simulink model "poco_ref_al_r307"  (Simulink 6.2)
settings: Solver=ode45  StartTime=0.0  StopTime=100000  RelTol=1e-3
libraries: xbsIndex_r3 x1012, xps_library x42, ddc_library x4, adcscope_lib x2, fft_library x2, pfb_library x2, delay_lib x1
(part 4 of 9)

== system poco_ref_al_r307/delay_wideband_prog0/delay_dp3 ==
  din : Inport  Port=1  LatchInput=off
  delay : Inport  Port=2  LatchInput=off
  AddSub : xbsIndex_r3/AddSub  mode=Subtraction  precision=User Defined  arith_type=Unsigned  n_bits=11  bin_pt=0  quantization=Truncate  overflow=Wrap  latency=1  explicit_period=off  period=1  use_carryin=off  use_carryout=off  en=off  dbl_ovrd=off  show_param=off  use_core=on  pipeline=off  use_rpm=on  gen_core=off
      settings: xl_area=[0, 0, 0, 0, 0, 0, 0]
  Constant2 : xbsIndex_r3/Constant  const=1  equ=P=C  arith_type=Boolean  n_bits=1  bin_pt=0  opselect=C  inp2=PCIN>>17  opr=+  inp1=P  carry=CIN  iostate=0  explicit_period=on  period=1  dbl_ovrd=off
  Constant4 : xbsIndex_r3/Constant  const=0  equ=P=C  arith_type=Boolean  n_bits=1  bin_pt=0  opselect=C  inp2=PCIN>>17  opr=+  inp1=P  carry=CIN  iostate=0  explicit_period=on  period=1  dbl_ovrd=off
  Dual Port RAM : S-Function  AncestorBlock=xbsIndex_r3/Dual Port RAM  FunctionName=xldpram  Parameters=sfcn_mwsv__  mask(Xilinx Dual Port Random Access Memory){depth=2048, initVector=0, write_mode_A=Read After Write, write_mode_B=Read After Write, latency=4, mem_collision=off, init_zero=on, explicit_period=off, period=1, dbl_ovrd=off, rst_a=off, init_a=0, rst_b=off, init_b=0, show_param=off, distributed_mem=off, use_rpm=off, gen_core=off, xl_area=[0, 0, 0, 0, 0, 0, 0], xl_use_area=off}
      mask prompts: initVector "Initial Value Vector"; write_mode_A "Write Mode:  Port A"; write_mode_B "Write Mode:  Port B"; mem_collision "Provide Output Valid Port"; init_zero "Zero Initial Output  (otherwise NaN)"; explicit_period "Use Explicit Sample Period"; period "Sample Period  (use -1 to inherit first known input period)"; dbl_ovrd "Override with Doubles"; rst_a "Provide Reset Port for Port A Output Register"; init_a "Initial Value for Port A Output Register"; rst_b "Provide Reset Port for Port B Output Register"; init_b "Initial Value for Port B Output Register"; show_param "---------------------- Show Implementation Parameters -----------------------------------------------------------------------------------"; distributed_mem "Use Distributed Memory (instead of block RAM)"; use_rpm "Use Placement Information for Core"; gen_core "Generate Core"; xl_area "FPGA Area [Slices, FFs, BRAMs, LUTs, IOBs, Emb. Mults, TBUFs]"; xl_use_area "Use Area Above For Estimation"
      mask help: Dual port random access memory (RAM). Independent address, data and write enable ports allow shared access to a single memory space. Dual ports enable simultaneous access to the memory space at different sample rates using multiple data widths.
      mask init: same as poco_ref_al_r307/delay_wideband_prog0/delay_dp/Dual Port RAM
      mask Help: eval('xlWeb(xlhtmldoclink(''Dual Port RAM''))');
      mask StyleString: edit,edit,popup(Read After Write|Read Before Write|No Read On Write),popup(Read After Write|Read Before Write|No Read On Write),edit,checkbox,checkbox,checkbox,edit,checkbox,checkbox,edit,checkbox,edit,checkbox,checkbox,checkbox,checkbox,edit,checkbox
      mask CallbackString: |||||||xldpramCallback|||xldpramCallback||xldpramCallback||xldpramCallback|xldpramCallback||||
      mask Display:
      | patch([0 iWidth iWidth 0],[0 0 iHeight iHeight] ,bg);
      | patch([0 iWidth iWidth 0],[iCy-2 iCy-2 iCy+2 iCy+2] , .9* bg);
      | patch(logoX,logoY , fg);
      | port_label('input',1,'addr_A');
      | port_label('input',2,'data_A');
      | port_label('input',3,'we_A');
      | port_label('input',4,'addr_B');
      | port_label('input',dataBPNum,dataBStr);
      | port_label('input',weBPNum,weBStr);
      | port_label('input',rstAPNum,rstAStr);
      | port_label('input',rstBPNum,rstBStr);
      | port_label('output',1,'A');
      | port_label('output',doutBPNum,'B');
      | port_label('output',voutAPNum,voutAStr);
      | port_label('output',voutBPNum,voutBStr);
      | ;plot([0 0 iWidth iWidth 0], [0 iHeight iHeight 0 0]);
  wr_addr : xbsIndex_r3/Counter  cnt_type=Free Running  n_bits=11  bin_pt=0  arith_type=Unsigned  start_count=0  cnt_to=Inf  cnt_by_val=1  operation=Up  explicit_period=off  period=1  load_pin=off  rst=off  en=off  dbl_ovrd=off  show_param=off  use_rpm=on  gen_core=off
      settings: xl_area=[0, 0, 0, 0, 0, 0, 0]
  dout : Outport
  wires:
  wr_addr/1 -> AddSub/1, Dual Port RAM/1
  Constant2/1 -> Dual Port RAM/3
  din/1 -> Dual Port RAM/5, Dual Port RAM/2
  Constant4/1 -> Dual Port RAM/6
  delay/1 -> AddSub/2
  AddSub/1 -> Dual Port RAM/4
  Dual Port RAM/2 -> dout/1

== system poco_ref_al_r307/delay_wideband_prog0/sync_delay ==
  In : Inport  Port=1  LatchInput=off
  Constant : xbsIndex_r3/Constant  const=1  equ=P=C  arith_type=Unsigned  n_bits=BitWidth  bin_pt=0  opselect=C  inp2=PCIN>>17  opr=+  inp1=P  carry=CIN  iostate=0  explicit_period=on  period=1  dbl_ovrd=off
  Constant1 : xbsIndex_r3/Constant  const=0  equ=P=C  arith_type=Unsigned  n_bits=BitWidth  bin_pt=0  opselect=C  inp2=PCIN>>17  opr=+  inp1=P  carry=CIN  iostate=0  explicit_period=on  period=1  dbl_ovrd=off
  Constant2 : xbsIndex_r3/Constant  const=DelayLen  equ=P=C  arith_type=Unsigned  n_bits=BitWidth  bin_pt=0  opselect=C  inp2=PCIN>>17  opr=+  inp1=P  carry=CIN  iostate=0  explicit_period=on  period=1  dbl_ovrd=off
  Constant3 : xbsIndex_r3/Constant  const=UseCounter  equ=P=C  arith_type=Unsigned  n_bits=1  bin_pt=0  opselect=C  inp2=PCIN>>17  opr=+  inp1=P  carry=CIN  iostate=0  explicit_period=on  period=1  dbl_ovrd=off
  Counter : xbsIndex_r3/Counter  cnt_type=Free Running  n_bits=BitWidth  bin_pt=0  arith_type=Unsigned  start_count=0  cnt_to=Inf  cnt_by_val=1  operation=Down  explicit_period=on  period=1  load_pin=on  rst=off  en=on  dbl_ovrd=off  show_param=off  use_rpm=on  gen_core=off
      settings: xl_area=[0, 0, 0, 0, 0, 0, 0]
  Logical : xbsIndex_r3/Logical  logical_function=OR  inputs=2  precision=Full  arith_type=Unsigned  n_bits=8  bin_pt=2  align_bp=on  latency=0  explicit_period=on  period=1  en=off  dbl_ovrd=off  show_param=off
      settings: xl_area=[0, 0, 0, 0, 0, 0, 0]
  Mux : xbsIndex_r3/Mux  inputs=2  precision=Full  arith_type="Signed  (2's comp)"  n_bits=8  bin_pt=2  quantization=Truncate  overflow=Wrap  latency=0  explicit_period=off  period=1  en=off  dbl_ovrd=off  show_param=off  mux_type=off  use_rpm=off  gen_core=off
      settings: xl_area=[0, 0, 0, 0, 0, 0, 0]
  Relational : xbsIndex_r3/Relational  mode=a=b  latency=0  explicit_period=off  period=1  en=off  dbl_ovrd=off  show_param=off
      settings: xl_area=[0, 0, 0, 0, 0, 0, 0]
  Relational1 : xbsIndex_r3/Relational  mode=a!=b  latency=0  explicit_period=on  period=1  en=off  dbl_ovrd=off  show_param=off
      settings: xl_area=[0, 0, 0, 0, 0, 0, 0]
  Out : Outport
  wires:
  Counter/1 -> Relational1/1, Relational/2
  Constant1/1 -> Relational1/2
  Constant/1 -> Relational/1
  Constant2/1 -> Counter/2
  In/1 -> Counter/1, Logical/1, Mux/2
  Logical/1 -> Counter/3
  Relational1/1 -> Logical/2
  Relational/1 -> Mux/3
  Constant3/1 -> Mux/1
  Mux/1 -> Out/1

== system poco_ref_al_r307/delay_wideband_prog1/barrel_switcher ==
  sel : Inport  Port=1  LatchInput=off
  sync_in : Inport  Port=2  LatchInput=off
  In1 : Inport  Port=3  LatchInput=off
  In2 : Inport  Port=4  LatchInput=off
  In3 : Inport  Port=5  LatchInput=off
  In4 : Inport  Port=6  LatchInput=off
  Delay1 : xbsIndex_r3/Delay  latency=1  reg_retiming=off  explicit_period=off  period=1  en=off  accept_only_valid=off  init_zero=on  dbl_ovrd=off  show_param=off
      settings: xl_area=[0, 0, 0, 0, 0, 0, 0]
  Delay_sync : xbsIndex_r3/Delay  latency=2  reg_retiming=off  explicit_period=off  period=1  en=off  accept_only_valid=off  init_zero=on  dbl_ovrd=off  show_param=off
      settings: xl_area=[0, 0, 0, 0, 0, 0, 0]
  Mux{11..12,21..22,31..32,41..42} (8 alike) : xbsIndex_r3/Mux  inputs=2  precision=Full  arith_type="Signed  (2's comp)"  n_bits=8  bin_pt=2  quantization=Truncate  overflow=Wrap  latency=1  explicit_period=off  period=1  en=off  dbl_ovrd=off  show_param=off  mux_type=off  use_rpm=off  gen_core=off
      settings: xl_area=[0, 0, 0, 0, 0, 0, 0]
  Slice1 : xbsIndex_r3/Slice  mode=Upper Bit Location + Width  nbits=1  bit1=-0  base1=MSB of Input  bit0=0  base0=LSB of Input  boolean_output=off  explicit_period=off  period=1  dbl_ovrd=off
  Slice2 : xbsIndex_r3/Slice  mode=Upper Bit Location + Width  nbits=1  bit1=-1  base1=MSB of Input  bit0=0  base0=LSB of Input  boolean_output=off  explicit_period=off  period=1  dbl_ovrd=off
  sync_out : Outport
  Out1 : Outport  Port=2
  Out2 : Outport  Port=3
  Out3 : Outport  Port=4
  Out4 : Outport  Port=5
  wires:
  Mux41/1 -> Mux32/3, Mux42/2
  Mux31/1 -> Mux22/3, Mux32/2
  Mux21/1 -> Mux12/3, Mux22/2
  Mux11/1 -> Mux42/3, Mux12/2
  Mux42/1 -> Out4/1
  In4/1 -> Mux21/3, Mux41/2
  Mux32/1 -> Out3/1
  In3/1 -> Mux11/3, Mux31/2
  Mux22/1 -> Out2/1
  In2/1 -> Mux41/3, Mux21/2
  Mux12/1 -> Out1/1
  In1/1 -> Mux31/3, Mux11/2
  Slice2/1 -> Mux42/1, Mux32/1, Mux22/1, Mux12/1
  Slice1/1 -> Mux41/1, Mux31/1, Mux21/1, Mux11/1
  Delay1/1 -> Slice2/1
  sel/1 -> Delay1/1, Slice1/1
  Delay_sync/1 -> sync_out/1
  sync_in/1 -> Delay_sync/1

== system poco_ref_al_r307/delay_wideband_prog1/delay_dp ==
  din : Inport  Port=1  LatchInput=off
  delay : Inport  Port=2  LatchInput=off
  AddSub : xbsIndex_r3/AddSub  mode=Subtraction  precision=User Defined  arith_type=Unsigned  n_bits=11  bin_pt=0  quantization=Truncate  overflow=Wrap  latency=1  explicit_period=off  period=1  use_carryin=off  use_carryout=off  en=off  dbl_ovrd=off  show_param=off  use_core=on  pipeline=off  use_rpm=on  gen_core=off
      settings: xl_area=[0, 0, 0, 0, 0, 0, 0]
  Constant2 : xbsIndex_r3/Constant  const=1  equ=P=C  arith_type=Boolean  n_bits=1  bin_pt=0  opselect=C  inp2=PCIN>>17  opr=+  inp1=P  carry=CIN  iostate=0  explicit_period=on  period=1  dbl_ovrd=off
  Constant4 : xbsIndex_r3/Constant  const=0  equ=P=C  arith_type=Boolean  n_bits=1  bin_pt=0  opselect=C  inp2=PCIN>>17  opr=+  inp1=P  carry=CIN  iostate=0  explicit_period=on  period=1  dbl_ovrd=off
  Dual Port RAM : S-Function  AncestorBlock=xbsIndex_r3/Dual Port RAM  FunctionName=xldpram  Parameters=sfcn_mwsv__  mask(Xilinx Dual Port Random Access Memory){depth=2048, initVector=0, write_mode_A=Read After Write, write_mode_B=Read After Write, latency=4, mem_collision=off, init_zero=on, explicit_period=off, period=1, dbl_ovrd=off, rst_a=off, init_a=0, rst_b=off, init_b=0, show_param=off, distributed_mem=off, use_rpm=off, gen_core=off, xl_area=[0, 0, 0, 0, 0, 0, 0], xl_use_area=off}
      mask prompts: initVector "Initial Value Vector"; write_mode_A "Write Mode:  Port A"; write_mode_B "Write Mode:  Port B"; mem_collision "Provide Output Valid Port"; init_zero "Zero Initial Output  (otherwise NaN)"; explicit_period "Use Explicit Sample Period"; period "Sample Period  (use -1 to inherit first known input period)"; dbl_ovrd "Override with Doubles"; rst_a "Provide Reset Port for Port A Output Register"; init_a "Initial Value for Port A Output Register"; rst_b "Provide Reset Port for Port B Output Register"; init_b "Initial Value for Port B Output Register"; show_param "---------------------- Show Implementation Parameters -----------------------------------------------------------------------------------"; distributed_mem "Use Distributed Memory (instead of block RAM)"; use_rpm "Use Placement Information for Core"; gen_core "Generate Core"; xl_area "FPGA Area [Slices, FFs, BRAMs, LUTs, IOBs, Emb. Mults, TBUFs]"; xl_use_area "Use Area Above For Estimation"
      mask help: Dual port random access memory (RAM). Independent address, data and write enable ports allow shared access to a single memory space. Dual ports enable simultaneous access to the memory space at different sample rates using multiple data widths.
      mask init: same as poco_ref_al_r307/delay_wideband_prog0/delay_dp/Dual Port RAM
      mask Help: eval('xlWeb(xlhtmldoclink(''Dual Port RAM''))');
      mask StyleString: edit,edit,popup(Read After Write|Read Before Write|No Read On Write),popup(Read After Write|Read Before Write|No Read On Write),edit,checkbox,checkbox,checkbox,edit,checkbox,checkbox,edit,checkbox,edit,checkbox,checkbox,checkbox,checkbox,edit,checkbox
      mask CallbackString: |||||||xldpramCallback|||xldpramCallback||xldpramCallback||xldpramCallback|xldpramCallback||||
      mask Display:
      | patch([0 iWidth iWidth 0],[0 0 iHeight iHeight] ,bg);
      | patch([0 iWidth iWidth 0],[iCy-2 iCy-2 iCy+2 iCy+2] , .9* bg);
      | patch(logoX,logoY , fg);
      | port_label('input',1,'addr_A');
      | port_label('input',2,'data_A');
      | port_label('input',3,'we_A');
      | port_label('input',4,'addr_B');
      | port_label('input',dataBPNum,dataBStr);
      | port_label('input',weBPNum,weBStr);
      | port_label('input',rstAPNum,rstAStr);
      | port_label('input',rstBPNum,rstBStr);
      | port_label('output',1,'A');
      | port_label('output',doutBPNum,'B');
      | port_label('output',voutAPNum,voutAStr);
      | port_label('output',voutBPNum,voutBStr);
      | ;plot([0 0 iWidth iWidth 0], [0 iHeight iHeight 0 0]);
  wr_addr : xbsIndex_r3/Counter  cnt_type=Free Running  n_bits=11  bin_pt=0  arith_type=Unsigned  start_count=0  cnt_to=Inf  cnt_by_val=1  operation=Up  explicit_period=off  period=1  load_pin=off  rst=off  en=off  dbl_ovrd=off  show_param=off  use_rpm=on  gen_core=off
      settings: xl_area=[0, 0, 0, 0, 0, 0, 0]
  dout : Outport
  wires:
  wr_addr/1 -> AddSub/1, Dual Port RAM/1
  Constant2/1 -> Dual Port RAM/3
  din/1 -> Dual Port RAM/5, Dual Port RAM/2
  Constant4/1 -> Dual Port RAM/6
  delay/1 -> AddSub/2
  AddSub/1 -> Dual Port RAM/4
  Dual Port RAM/2 -> dout/1

== system poco_ref_al_r307/delay_wideband_prog1/delay_dp1 ==
  din : Inport  Port=1  LatchInput=off
  delay : Inport  Port=2  LatchInput=off
  AddSub : xbsIndex_r3/AddSub  mode=Subtraction  precision=User Defined  arith_type=Unsigned  n_bits=11  bin_pt=0  quantization=Truncate  overflow=Wrap  latency=1  explicit_period=off  period=1  use_carryin=off  use_carryout=off  en=off  dbl_ovrd=off  show_param=off  use_core=on  pipeline=off  use_rpm=on  gen_core=off
      settings: xl_area=[0, 0, 0, 0, 0, 0, 0]
  Constant2 : xbsIndex_r3/Constant  const=1  equ=P=C  arith_type=Boolean  n_bits=1  bin_pt=0  opselect=C  inp2=PCIN>>17  opr=+  inp1=P  carry=CIN  iostate=0  explicit_period=on  period=1  dbl_ovrd=off
  Constant4 : xbsIndex_r3/Constant  const=0  equ=P=C  arith_type=Boolean  n_bits=1  bin_pt=0  opselect=C  inp2=PCIN>>17  opr=+  inp1=P  carry=CIN  iostate=0  explicit_period=on  period=1  dbl_ovrd=off
  Dual Port RAM : S-Function  AncestorBlock=xbsIndex_r3/Dual Port RAM  FunctionName=xldpram  Parameters=sfcn_mwsv__  mask(Xilinx Dual Port Random Access Memory){depth=2048, initVector=0, write_mode_A=Read After Write, write_mode_B=Read After Write, latency=4, mem_collision=off, init_zero=on, explicit_period=off, period=1, dbl_ovrd=off, rst_a=off, init_a=0, rst_b=off, init_b=0, show_param=off, distributed_mem=off, use_rpm=off, gen_core=off, xl_area=[0, 0, 0, 0, 0, 0, 0], xl_use_area=off}
      mask prompts: initVector "Initial Value Vector"; write_mode_A "Write Mode:  Port A"; write_mode_B "Write Mode:  Port B"; mem_collision "Provide Output Valid Port"; init_zero "Zero Initial Output  (otherwise NaN)"; explicit_period "Use Explicit Sample Period"; period "Sample Period  (use -1 to inherit first known input period)"; dbl_ovrd "Override with Doubles"; rst_a "Provide Reset Port for Port A Output Register"; init_a "Initial Value for Port A Output Register"; rst_b "Provide Reset Port for Port B Output Register"; init_b "Initial Value for Port B Output Register"; show_param "---------------------- Show Implementation Parameters -----------------------------------------------------------------------------------"; distributed_mem "Use Distributed Memory (instead of block RAM)"; use_rpm "Use Placement Information for Core"; gen_core "Generate Core"; xl_area "FPGA Area [Slices, FFs, BRAMs, LUTs, IOBs, Emb. Mults, TBUFs]"; xl_use_area "Use Area Above For Estimation"
      mask help: Dual port random access memory (RAM). Independent address, data and write enable ports allow shared access to a single memory space. Dual ports enable simultaneous access to the memory space at different sample rates using multiple data widths.
      mask init: same as poco_ref_al_r307/delay_wideband_prog0/delay_dp/Dual Port RAM
      mask Help: eval('xlWeb(xlhtmldoclink(''Dual Port RAM''))');
      mask StyleString: edit,edit,popup(Read After Write|Read Before Write|No Read On Write),popup(Read After Write|Read Before Write|No Read On Write),edit,checkbox,checkbox,checkbox,edit,checkbox,checkbox,edit,checkbox,edit,checkbox,checkbox,checkbox,checkbox,edit,checkbox
      mask CallbackString: |||||||xldpramCallback|||xldpramCallback||xldpramCallback||xldpramCallback|xldpramCallback||||
      mask Display:
      | patch([0 iWidth iWidth 0],[0 0 iHeight iHeight] ,bg);
      | patch([0 iWidth iWidth 0],[iCy-2 iCy-2 iCy+2 iCy+2] , .9* bg);
      | patch(logoX,logoY , fg);
      | port_label('input',1,'addr_A');
      | port_label('input',2,'data_A');
      | port_label('input',3,'we_A');
      | port_label('input',4,'addr_B');
      | port_label('input',dataBPNum,dataBStr);
      | port_label('input',weBPNum,weBStr);
      | port_label('input',rstAPNum,rstAStr);
      | port_label('input',rstBPNum,rstBStr);
      | port_label('output',1,'A');
      | port_label('output',doutBPNum,'B');
      | port_label('output',voutAPNum,voutAStr);
      | port_label('output',voutBPNum,voutBStr);
      | ;plot([0 0 iWidth iWidth 0], [0 iHeight iHeight 0 0]);
  wr_addr : xbsIndex_r3/Counter  cnt_type=Free Running  n_bits=11  bin_pt=0  arith_type=Unsigned  start_count=0  cnt_to=Inf  cnt_by_val=1  operation=Up  explicit_period=off  period=1  load_pin=off  rst=off  en=off  dbl_ovrd=off  show_param=off  use_rpm=on  gen_core=off
      settings: xl_area=[0, 0, 0, 0, 0, 0, 0]
  dout : Outport
  wires:
  Dual Port RAM/2 -> dout/1
  AddSub/1 -> Dual Port RAM/4
  delay/1 -> AddSub/2
  Constant4/1 -> Dual Port RAM/6
  din/1 -> Dual Port RAM/2, Dual Port RAM/5
  Constant2/1 -> Dual Port RAM/3
  wr_addr/1 -> Dual Port RAM/1, AddSub/1

== system poco_ref_al_r307/delay_wideband_prog1/delay_dp2 ==
  din : Inport  Port=1  LatchInput=off
  delay : Inport  Port=2  LatchInput=off
  AddSub : xbsIndex_r3/AddSub  mode=Subtraction  precision=User Defined  arith_type=Unsigned  n_bits=11  bin_pt=0  quantization=Truncate  overflow=Wrap  latency=1  explicit_period=off  period=1  use_carryin=off  use_carryout=off  en=off  dbl_ovrd=off  show_param=off  use_core=on  pipeline=off  use_rpm=on  gen_core=off
      settings: xl_area=[0, 0, 0, 0, 0, 0, 0]
  Constant2 : xbsIndex_r3/Constant  const=1  equ=P=C  arith_type=Boolean  n_bits=1  bin_pt=0  opselect=C  inp2=PCIN>>17  opr=+  inp1=P  carry=CIN  iostate=0  explicit_period=on  period=1  dbl_ovrd=off
  Constant4 : xbsIndex_r3/Constant  const=0  equ=P=C  arith_type=Boolean  n_bits=1  bin_pt=0  opselect=C  inp2=PCIN>>17  opr=+  inp1=P  carry=CIN  iostate=0  explicit_period=on  period=1  dbl_ovrd=off
  Dual Port RAM : S-Function  AncestorBlock=xbsIndex_r3/Dual Port RAM  FunctionName=xldpram  Parameters=sfcn_mwsv__  mask(Xilinx Dual Port Random Access Memory){depth=2048, initVector=0, write_mode_A=Read After Write, write_mode_B=Read After Write, latency=4, mem_collision=off, init_zero=on, explicit_period=off, period=1, dbl_ovrd=off, rst_a=off, init_a=0, rst_b=off, init_b=0, show_param=off, distributed_mem=off, use_rpm=off, gen_core=off, xl_area=[0, 0, 0, 0, 0, 0, 0], xl_use_area=off}
      mask prompts: initVector "Initial Value Vector"; write_mode_A "Write Mode:  Port A"; write_mode_B "Write Mode:  Port B"; mem_collision "Provide Output Valid Port"; init_zero "Zero Initial Output  (otherwise NaN)"; explicit_period "Use Explicit Sample Period"; period "Sample Period  (use -1 to inherit first known input period)"; dbl_ovrd "Override with Doubles"; rst_a "Provide Reset Port for Port A Output Register"; init_a "Initial Value for Port A Output Register"; rst_b "Provide Reset Port for Port B Output Register"; init_b "Initial Value for Port B Output Register"; show_param "---------------------- Show Implementation Parameters -----------------------------------------------------------------------------------"; distributed_mem "Use Distributed Memory (instead of block RAM)"; use_rpm "Use Placement Information for Core"; gen_core "Generate Core"; xl_area "FPGA Area [Slices, FFs, BRAMs, LUTs, IOBs, Emb. Mults, TBUFs]"; xl_use_area "Use Area Above For Estimation"
      mask help: Dual port random access memory (RAM). Independent address, data and write enable ports allow shared access to a single memory space. Dual ports enable simultaneous access to the memory space at different sample rates using multiple data widths.
      mask init: same as poco_ref_al_r307/delay_wideband_prog0/delay_dp/Dual Port RAM
      mask Help: eval('xlWeb(xlhtmldoclink(''Dual Port RAM''))');
      mask StyleString: edit,edit,popup(Read After Write|Read Before Write|No Read On Write),popup(Read After Write|Read Before Write|No Read On Write),edit,checkbox,checkbox,checkbox,edit,checkbox,checkbox,edit,checkbox,edit,checkbox,checkbox,checkbox,checkbox,edit,checkbox
      mask CallbackString: |||||||xldpramCallback|||xldpramCallback||xldpramCallback||xldpramCallback|xldpramCallback||||
      mask Display:
      | patch([0 iWidth iWidth 0],[0 0 iHeight iHeight] ,bg);
      | patch([0 iWidth iWidth 0],[iCy-2 iCy-2 iCy+2 iCy+2] , .9* bg);
      | patch(logoX,logoY , fg);
      | port_label('input',1,'addr_A');
      | port_label('input',2,'data_A');
      | port_label('input',3,'we_A');
      | port_label('input',4,'addr_B');
      | port_label('input',dataBPNum,dataBStr);
      | port_label('input',weBPNum,weBStr);
      | port_label('input',rstAPNum,rstAStr);
      | port_label('input',rstBPNum,rstBStr);
      | port_label('output',1,'A');
      | port_label('output',doutBPNum,'B');
      | port_label('output',voutAPNum,voutAStr);
      | port_label('output',voutBPNum,voutBStr);
      | ;plot([0 0 iWidth iWidth 0], [0 iHeight iHeight 0 0]);
  wr_addr : xbsIndex_r3/Counter  cnt_type=Free Running  n_bits=11  bin_pt=0  arith_type=Unsigned  start_count=0  cnt_to=Inf  cnt_by_val=1  operation=Up  explicit_period=off  period=1  load_pin=off  rst=off  en=off  dbl_ovrd=off  show_param=off  use_rpm=on  gen_core=off
      settings: xl_area=[0, 0, 0, 0, 0, 0, 0]
  dout : Outport
  wires:
  wr_addr/1 -> AddSub/1, Dual Port RAM/1
  Constant2/1 -> Dual Port RAM/3
  din/1 -> Dual Port RAM/5, Dual Port RAM/2
  Constant4/1 -> Dual Port RAM/6
  delay/1 -> AddSub/2
  AddSub/1 -> Dual Port RAM/4
  Dual Port RAM/2 -> dout/1

== system poco_ref_al_r307/delay_wideband_prog1/delay_dp3 ==
  din : Inport  Port=1  LatchInput=off
  delay : Inport  Port=2  LatchInput=off
  AddSub : xbsIndex_r3/AddSub  mode=Subtraction  precision=User Defined  arith_type=Unsigned  n_bits=11  bin_pt=0  quantization=Truncate  overflow=Wrap  latency=1  explicit_period=off  period=1  use_carryin=off  use_carryout=off  en=off  dbl_ovrd=off  show_param=off  use_core=on  pipeline=off  use_rpm=on  gen_core=off
      settings: xl_area=[0, 0, 0, 0, 0, 0, 0]
  Constant2 : xbsIndex_r3/Constant  const=1  equ=P=C  arith_type=Boolean  n_bits=1  bin_pt=0  opselect=C  inp2=PCIN>>17  opr=+  inp1=P  carry=CIN  iostate=0  explicit_period=on  period=1  dbl_ovrd=off
  Constant4 : xbsIndex_r3/Constant  const=0  equ=P=C  arith_type=Boolean  n_bits=1  bin_pt=0  opselect=C  inp2=PCIN>>17  opr=+  inp1=P  carry=CIN  iostate=0  explicit_period=on  period=1  dbl_ovrd=off
  Dual Port RAM : S-Function  AncestorBlock=xbsIndex_r3/Dual Port RAM  FunctionName=xldpram  Parameters=sfcn_mwsv__  mask(Xilinx Dual Port Random Access Memory){depth=2048, initVector=0, write_mode_A=Read After Write, write_mode_B=Read After Write, latency=4, mem_collision=off, init_zero=on, explicit_period=off, period=1, dbl_ovrd=off, rst_a=off, init_a=0, rst_b=off, init_b=0, show_param=off, distributed_mem=off, use_rpm=off, gen_core=off, xl_area=[0, 0, 0, 0, 0, 0, 0], xl_use_area=off}
      mask prompts: initVector "Initial Value Vector"; write_mode_A "Write Mode:  Port A"; write_mode_B "Write Mode:  Port B"; mem_collision "Provide Output Valid Port"; init_zero "Zero Initial Output  (otherwise NaN)"; explicit_period "Use Explicit Sample Period"; period "Sample Period  (use -1 to inherit first known input period)"; dbl_ovrd "Override with Doubles"; rst_a "Provide Reset Port for Port A Output Register"; init_a "Initial Value for Port A Output Register"; rst_b "Provide Reset Port for Port B Output Register"; init_b "Initial Value for Port B Output Register"; show_param "---------------------- Show Implementation Parameters -----------------------------------------------------------------------------------"; distributed_mem "Use Distributed Memory (instead of block RAM)"; use_rpm "Use Placement Information for Core"; gen_core "Generate Core"; xl_area "FPGA Area [Slices, FFs, BRAMs, LUTs, IOBs, Emb. Mults, TBUFs]"; xl_use_area "Use Area Above For Estimation"
      mask help: Dual port random access memory (RAM). Independent address, data and write enable ports allow shared access to a single memory space. Dual ports enable simultaneous access to the memory space at different sample rates using multiple data widths.
      mask init: same as poco_ref_al_r307/delay_wideband_prog0/delay_dp/Dual Port RAM
      mask Help: eval('xlWeb(xlhtmldoclink(''Dual Port RAM''))');
      mask StyleString: edit,edit,popup(Read After Write|Read Before Write|No Read On Write),popup(Read After Write|Read Before Write|No Read On Write),edit,checkbox,checkbox,checkbox,edit,checkbox,checkbox,edit,checkbox,edit,checkbox,checkbox,checkbox,checkbox,edit,checkbox
      mask CallbackString: |||||||xldpramCallback|||xldpramCallback||xldpramCallback||xldpramCallback|xldpramCallback||||
      mask Display:
      | patch([0 iWidth iWidth 0],[0 0 iHeight iHeight] ,bg);
      | patch([0 iWidth iWidth 0],[iCy-2 iCy-2 iCy+2 iCy+2] , .9* bg);
      | patch(logoX,logoY , fg);
      | port_label('input',1,'addr_A');
      | port_label('input',2,'data_A');
      | port_label('input',3,'we_A');
      | port_label('input',4,'addr_B');
      | port_label('input',dataBPNum,dataBStr);
      | port_label('input',weBPNum,weBStr);
      | port_label('input',rstAPNum,rstAStr);
      | port_label('input',rstBPNum,rstBStr);
      | port_label('output',1,'A');
      | port_label('output',doutBPNum,'B');
      | port_label('output',voutAPNum,voutAStr);
      | port_label('output',voutBPNum,voutBStr);
      | ;plot([0 0 iWidth iWidth 0], [0 iHeight iHeight 0 0]);
  wr_addr : xbsIndex_r3/Counter  cnt_type=Free Running  n_bits=11  bin_pt=0  arith_type=Unsigned  start_count=0  cnt_to=Inf  cnt_by_val=1  operation=Up  explicit_period=off  period=1  load_pin=off  rst=off  en=off  dbl_ovrd=off  show_param=off  use_rpm=on  gen_core=off
      settings: xl_area=[0, 0, 0, 0, 0, 0, 0]
  dout : Outport
  wires:
  Dual Port RAM/2 -> dout/1
  AddSub/1 -> Dual Port RAM/4
  delay/1 -> AddSub/2
  Constant4/1 -> Dual Port RAM/6
  din/1 -> Dual Port RAM/2, Dual Port RAM/5
  Constant2/1 -> Dual Port RAM/3
  wr_addr/1 -> Dual Port RAM/1, AddSub/1

== system poco_ref_al_r307/delay_wideband_prog1/sync_delay ==
  In : Inport  Port=1  LatchInput=off
  Constant : xbsIndex_r3/Constant  const=1  equ=P=C  arith_type=Unsigned  n_bits=BitWidth  bin_pt=0  opselect=C  inp2=PCIN>>17  opr=+  inp1=P  carry=CIN  iostate=0  explicit_period=on  period=1  dbl_ovrd=off
  Constant1 : xbsIndex_r3/Constant  const=0  equ=P=C  arith_type=Unsigned  n_bits=BitWidth  bin_pt=0  opselect=C  inp2=PCIN>>17  opr=+  inp1=P  carry=CIN  iostate=0  explicit_period=on  period=1  dbl_ovrd=off
  Constant2 : xbsIndex_r3/Constant  const=DelayLen  equ=P=C  arith_type=Unsigned  n_bits=BitWidth  bin_pt=0  opselect=C  inp2=PCIN>>17  opr=+  inp1=P  carry=CIN  iostate=0  explicit_period=on  period=1  dbl_ovrd=off
  Constant3 : xbsIndex_r3/Constant  const=UseCounter  equ=P=C  arith_type=Unsigned  n_bits=1  bin_pt=0  opselect=C  inp2=PCIN>>17  opr=+  inp1=P  carry=CIN  iostate=0  explicit_period=on  period=1  dbl_ovrd=off
  Counter : xbsIndex_r3/Counter  cnt_type=Free Running  n_bits=BitWidth  bin_pt=0  arith_type=Unsigned  start_count=0  cnt_to=Inf  cnt_by_val=1  operation=Down  explicit_period=on  period=1  load_pin=on  rst=off  en=on  dbl_ovrd=off  show_param=off  use_rpm=on  gen_core=off
      settings: xl_area=[0, 0, 0, 0, 0, 0, 0]
  Logical : xbsIndex_r3/Logical  logical_function=OR  inputs=2  precision=Full  arith_type=Unsigned  n_bits=8  bin_pt=2  align_bp=on  latency=0  explicit_period=on  period=1  en=off  dbl_ovrd=off  show_param=off
      settings: xl_area=[0, 0, 0, 0, 0, 0, 0]
  Mux : xbsIndex_r3/Mux  inputs=2  precision=Full  arith_type="Signed  (2's comp)"  n_bits=8  bin_pt=2  quantization=Truncate  overflow=Wrap  latency=0  explicit_period=off  period=1  en=off  dbl_ovrd=off  show_param=off  mux_type=off  use_rpm=off  gen_core=off
      settings: xl_area=[0, 0, 0, 0, 0, 0, 0]
  Relational : xbsIndex_r3/Relational  mode=a=b  latency=0  explicit_period=off  period=1  en=off  dbl_ovrd=off  show_param=off
      settings: xl_area=[0, 0, 0, 0, 0, 0, 0]
  Relational1 : xbsIndex_r3/Relational  mode=a!=b  latency=0  explicit_period=on  period=1  en=off  dbl_ovrd=off  show_param=off
      settings: xl_area=[0, 0, 0, 0, 0, 0, 0]
  Out : Outport
  wires:
  Mux/1 -> Out/1
  Constant3/1 -> Mux/1
  Relational/1 -> Mux/3
  Relational1/1 -> Logical/2
  Logical/1 -> Counter/3
  In/1 -> Mux/2, Logical/1, Counter/1
  Constant2/1 -> Counter/2
  Constant/1 -> Relational/1
  Constant1/1 -> Relational1/2
  Counter/1 -> Relational/2, Relational1/1

== system poco_ref_al_r307/delay_wideband_prog2/barrel_switcher ==
  sel : Inport  Port=1  LatchInput=off
  sync_in : Inport  Port=2  LatchInput=off
  In1 : Inport  Port=3  LatchInput=off
  In2 : Inport  Port=4  LatchInput=off
  In3 : Inport  Port=5  LatchInput=off
  In4 : Inport  Port=6  LatchInput=off
  Delay1 : xbsIndex_r3/Delay  latency=1  reg_retiming=off  explicit_period=off  period=1  en=off  accept_only_valid=off  init_zero=on  dbl_ovrd=off  show_param=off
      settings: xl_area=[0, 0, 0, 0, 0, 0, 0]
  Delay_sync : xbsIndex_r3/Delay  latency=2  reg_retiming=off  explicit_period=off  period=1  en=off  accept_only_valid=off  init_zero=on  dbl_ovrd=off  show_param=off
      settings: xl_area=[0, 0, 0, 0, 0, 0, 0]
  Mux{11..12,21..22,31..32,41..42} (8 alike) : xbsIndex_r3/Mux  inputs=2  precision=Full  arith_type="Signed  (2's comp)"  n_bits=8  bin_pt=2  quantization=Truncate  overflow=Wrap  latency=1  explicit_period=off  period=1  en=off  dbl_ovrd=off  show_param=off  mux_type=off  use_rpm=off  gen_core=off
      settings: xl_area=[0, 0, 0, 0, 0, 0, 0]
  Slice1 : xbsIndex_r3/Slice  mode=Upper Bit Location + Width  nbits=1  bit1=-0  base1=MSB of Input  bit0=0  base0=LSB of Input  boolean_output=off  explicit_period=off  period=1  dbl_ovrd=off
  Slice2 : xbsIndex_r3/Slice  mode=Upper Bit Location + Width  nbits=1  bit1=-1  base1=MSB of Input  bit0=0  base0=LSB of Input  boolean_output=off  explicit_period=off  period=1  dbl_ovrd=off
  sync_out : Outport
  Out1 : Outport  Port=2
  Out2 : Outport  Port=3
  Out3 : Outport  Port=4
  Out4 : Outport  Port=5
  wires:
  sync_in/1 -> Delay_sync/1
  Delay_sync/1 -> sync_out/1
  sel/1 -> Slice1/1, Delay1/1
  Delay1/1 -> Slice2/1
  Slice1/1 -> Mux11/1, Mux21/1, Mux31/1, Mux41/1
  Slice2/1 -> Mux12/1, Mux22/1, Mux32/1, Mux42/1
  In1/1 -> Mux11/2, Mux31/3
  Mux12/1 -> Out1/1
  In2/1 -> Mux21/2, Mux41/3
  Mux22/1 -> Out2/1
  In3/1 -> Mux31/2, Mux11/3
  Mux32/1 -> Out3/1
  In4/1 -> Mux41/2, Mux21/3
  Mux42/1 -> Out4/1
  Mux11/1 -> Mux12/2, Mux42/3
  Mux21/1 -> Mux22/2, Mux12/3
  Mux31/1 -> Mux32/2, Mux22/3
  Mux41/1 -> Mux42/2, Mux32/3

== system poco_ref_al_r307/delay_wideband_prog2/delay_dp ==
  din : Inport  Port=1  LatchInput=off
  delay : Inport  Port=2  LatchInput=off
  AddSub : xbsIndex_r3/AddSub  mode=Subtraction  precision=User Defined  arith_type=Unsigned  n_bits=11  bin_pt=0  quantization=Truncate  overflow=Wrap  latency=1  explicit_period=off  period=1  use_carryin=off  use_carryout=off  en=off  dbl_ovrd=off  show_param=off  use_core=on  pipeline=off  use_rpm=on  gen_core=off
      settings: xl_area=[0, 0, 0, 0, 0, 0, 0]
  Constant2 : xbsIndex_r3/Constant  const=1  equ=P=C  arith_type=Boolean  n_bits=1  bin_pt=0  opselect=C  inp2=PCIN>>17  opr=+  inp1=P  carry=CIN  iostate=0  explicit_period=on  period=1  dbl_ovrd=off
  Constant4 : xbsIndex_r3/Constant  const=0  equ=P=C  arith_type=Boolean  n_bits=1  bin_pt=0  opselect=C  inp2=PCIN>>17  opr=+  inp1=P  carry=CIN  iostate=0  explicit_period=on  period=1  dbl_ovrd=off
  Dual Port RAM : S-Function  AncestorBlock=xbsIndex_r3/Dual Port RAM  FunctionName=xldpram  Parameters=sfcn_mwsv__  mask(Xilinx Dual Port Random Access Memory){depth=2048, initVector=0, write_mode_A=Read After Write, write_mode_B=Read After Write, latency=4, mem_collision=off, init_zero=on, explicit_period=off, period=1, dbl_ovrd=off, rst_a=off, init_a=0, rst_b=off, init_b=0, show_param=off, distributed_mem=off, use_rpm=off, gen_core=off, xl_area=[0, 0, 0, 0, 0, 0, 0], xl_use_area=off}
      mask prompts: initVector "Initial Value Vector"; write_mode_A "Write Mode:  Port A"; write_mode_B "Write Mode:  Port B"; mem_collision "Provide Output Valid Port"; init_zero "Zero Initial Output  (otherwise NaN)"; explicit_period "Use Explicit Sample Period"; period "Sample Period  (use -1 to inherit first known input period)"; dbl_ovrd "Override with Doubles"; rst_a "Provide Reset Port for Port A Output Register"; init_a "Initial Value for Port A Output Register"; rst_b "Provide Reset Port for Port B Output Register"; init_b "Initial Value for Port B Output Register"; show_param "---------------------- Show Implementation Parameters -----------------------------------------------------------------------------------"; distributed_mem "Use Distributed Memory (instead of block RAM)"; use_rpm "Use Placement Information for Core"; gen_core "Generate Core"; xl_area "FPGA Area [Slices, FFs, BRAMs, LUTs, IOBs, Emb. Mults, TBUFs]"; xl_use_area "Use Area Above For Estimation"
      mask help: Dual port random access memory (RAM). Independent address, data and write enable ports allow shared access to a single memory space. Dual ports enable simultaneous access to the memory space at different sample rates using multiple data widths.
      mask init: same as poco_ref_al_r307/delay_wideband_prog0/delay_dp/Dual Port RAM
      mask Help: eval('xlWeb(xlhtmldoclink(''Dual Port RAM''))');
      mask StyleString: edit,edit,popup(Read After Write|Read Before Write|No Read On Write),popup(Read After Write|Read Before Write|No Read On Write),edit,checkbox,checkbox,checkbox,edit,checkbox,checkbox,edit,checkbox,edit,checkbox,checkbox,checkbox,checkbox,edit,checkbox
      mask CallbackString: |||||||xldpramCallback|||xldpramCallback||xldpramCallback||xldpramCallback|xldpramCallback||||
      mask Display:
      | patch([0 iWidth iWidth 0],[0 0 iHeight iHeight] ,bg);
      | patch([0 iWidth iWidth 0],[iCy-2 iCy-2 iCy+2 iCy+2] , .9* bg);
      | patch(logoX,logoY , fg);
      | port_label('input',1,'addr_A');
      | port_label('input',2,'data_A');
      | port_label('input',3,'we_A');
      | port_label('input',4,'addr_B');
      | port_label('input',dataBPNum,dataBStr);
      | port_label('input',weBPNum,weBStr);
      | port_label('input',rstAPNum,rstAStr);
      | port_label('input',rstBPNum,rstBStr);
      | port_label('output',1,'A');
      | port_label('output',doutBPNum,'B');
      | port_label('output',voutAPNum,voutAStr);
      | port_label('output',voutBPNum,voutBStr);
      | ;plot([0 0 iWidth iWidth 0], [0 iHeight iHeight 0 0]);
  wr_addr : xbsIndex_r3/Counter  cnt_type=Free Running  n_bits=11  bin_pt=0  arith_type=Unsigned  start_count=0  cnt_to=Inf  cnt_by_val=1  operation=Up  explicit_period=off  period=1  load_pin=off  rst=off  en=off  dbl_ovrd=off  show_param=off  use_rpm=on  gen_core=off
      settings: xl_area=[0, 0, 0, 0, 0, 0, 0]
  dout : Outport
  wires:
  Dual Port RAM/2 -> dout/1
  AddSub/1 -> Dual Port RAM/4
  delay/1 -> AddSub/2
  Constant4/1 -> Dual Port RAM/6
  din/1 -> Dual Port RAM/2, Dual Port RAM/5
  Constant2/1 -> Dual Port RAM/3
  wr_addr/1 -> Dual Port RAM/1, AddSub/1

== system poco_ref_al_r307/delay_wideband_prog2/delay_dp1 ==
  din : Inport  Port=1  LatchInput=off
  delay : Inport  Port=2  LatchInput=off
  AddSub : xbsIndex_r3/AddSub  mode=Subtraction  precision=User Defined  arith_type=Unsigned  n_bits=11  bin_pt=0  quantization=Truncate  overflow=Wrap  latency=1  explicit_period=off  period=1  use_carryin=off  use_carryout=off  en=off  dbl_ovrd=off  show_param=off  use_core=on  pipeline=off  use_rpm=on  gen_core=off
      settings: xl_area=[0, 0, 0, 0, 0, 0, 0]
  Constant2 : xbsIndex_r3/Constant  const=1  equ=P=C  arith_type=Boolean  n_bits=1  bin_pt=0  opselect=C  inp2=PCIN>>17  opr=+  inp1=P  carry=CIN  iostate=0  explicit_period=on  period=1  dbl_ovrd=off
  Constant4 : xbsIndex_r3/Constant  const=0  equ=P=C  arith_type=Boolean  n_bits=1  bin_pt=0  opselect=C  inp2=PCIN>>17  opr=+  inp1=P  carry=CIN  iostate=0  explicit_period=on  period=1  dbl_ovrd=off
  Dual Port RAM : S-Function  AncestorBlock=xbsIndex_r3/Dual Port RAM  FunctionName=xldpram  Parameters=sfcn_mwsv__  mask(Xilinx Dual Port Random Access Memory){depth=2048, initVector=0, write_mode_A=Read After Write, write_mode_B=Read After Write, latency=4, mem_collision=off, init_zero=on, explicit_period=off, period=1, dbl_ovrd=off, rst_a=off, init_a=0, rst_b=off, init_b=0, show_param=off, distributed_mem=off, use_rpm=off, gen_core=off, xl_area=[0, 0, 0, 0, 0, 0, 0], xl_use_area=off}
      mask prompts: initVector "Initial Value Vector"; write_mode_A "Write Mode:  Port A"; write_mode_B "Write Mode:  Port B"; mem_collision "Provide Output Valid Port"; init_zero "Zero Initial Output  (otherwise NaN)"; explicit_period "Use Explicit Sample Period"; period "Sample Period  (use -1 to inherit first known input period)"; dbl_ovrd "Override with Doubles"; rst_a "Provide Reset Port for Port A Output Register"; init_a "Initial Value for Port A Output Register"; rst_b "Provide Reset Port for Port B Output Register"; init_b "Initial Value for Port B Output Register"; show_param "---------------------- Show Implementation Parameters -----------------------------------------------------------------------------------"; distributed_mem "Use Distributed Memory (instead of block RAM)"; use_rpm "Use Placement Information for Core"; gen_core "Generate Core"; xl_area "FPGA Area [Slices, FFs, BRAMs, LUTs, IOBs, Emb. Mults, TBUFs]"; xl_use_area "Use Area Above For Estimation"
      mask help: Dual port random access memory (RAM). Independent address, data and write enable ports allow shared access to a single memory space. Dual ports enable simultaneous access to the memory space at different sample rates using multiple data widths.
      mask init: same as poco_ref_al_r307/delay_wideband_prog0/delay_dp/Dual Port RAM
      mask Help: eval('xlWeb(xlhtmldoclink(''Dual Port RAM''))');
      mask StyleString: edit,edit,popup(Read After Write|Read Before Write|No Read On Write),popup(Read After Write|Read Before Write|No Read On Write),edit,checkbox,checkbox,checkbox,edit,checkbox,checkbox,edit,checkbox,edit,checkbox,checkbox,checkbox,checkbox,edit,checkbox
      mask CallbackString: |||||||xldpramCallback|||xldpramCallback||xldpramCallback||xldpramCallback|xldpramCallback||||
      mask Display:
      | patch([0 iWidth iWidth 0],[0 0 iHeight iHeight] ,bg);
      | patch([0 iWidth iWidth 0],[iCy-2 iCy-2 iCy+2 iCy+2] , .9* bg);
      | patch(logoX,logoY , fg);
      | port_label('input',1,'addr_A');
      | port_label('input',2,'data_A');
      | port_label('input',3,'we_A');
      | port_label('input',4,'addr_B');
      | port_label('input',dataBPNum,dataBStr);
      | port_label('input',weBPNum,weBStr);
      | port_label('input',rstAPNum,rstAStr);
      | port_label('input',rstBPNum,rstBStr);
      | port_label('output',1,'A');
      | port_label('output',doutBPNum,'B');
      | port_label('output',voutAPNum,voutAStr);
      | port_label('output',voutBPNum,voutBStr);
      | ;plot([0 0 iWidth iWidth 0], [0 iHeight iHeight 0 0]);
  wr_addr : xbsIndex_r3/Counter  cnt_type=Free Running  n_bits=11  bin_pt=0  arith_type=Unsigned  start_count=0  cnt_to=Inf  cnt_by_val=1  operation=Up  explicit_period=off  period=1  load_pin=off  rst=off  en=off  dbl_ovrd=off  show_param=off  use_rpm=on  gen_core=off
      settings: xl_area=[0, 0, 0, 0, 0, 0, 0]
  dout : Outport
  wires:
  wr_addr/1 -> AddSub/1, Dual Port RAM/1
  Constant2/1 -> Dual Port RAM/3
  din/1 -> Dual Port RAM/5, Dual Port RAM/2
  Constant4/1 -> Dual Port RAM/6
  delay/1 -> AddSub/2
  AddSub/1 -> Dual Port RAM/4
  Dual Port RAM/2 -> dout/1

== system poco_ref_al_r307/delay_wideband_prog2/delay_dp2 ==
  din : Inport  Port=1  LatchInput=off
  delay : Inport  Port=2  LatchInput=off
  AddSub : xbsIndex_r3/AddSub  mode=Subtraction  precision=User Defined  arith_type=Unsigned  n_bits=11  bin_pt=0  quantization=Truncate  overflow=Wrap  latency=1  explicit_period=off  period=1  use_carryin=off  use_carryout=off  en=off  dbl_ovrd=off  show_param=off  use_core=on  pipeline=off  use_rpm=on  gen_core=off
      settings: xl_area=[0, 0, 0, 0, 0, 0, 0]
  Constant2 : xbsIndex_r3/Constant  const=1  equ=P=C  arith_type=Boolean  n_bits=1  bin_pt=0  opselect=C  inp2=PCIN>>17  opr=+  inp1=P  carry=CIN  iostate=0  explicit_period=on  period=1  dbl_ovrd=off
  Constant4 : xbsIndex_r3/Constant  const=0  equ=P=C  arith_type=Boolean  n_bits=1  bin_pt=0  opselect=C  inp2=PCIN>>17  opr=+  inp1=P  carry=CIN  iostate=0  explicit_period=on  period=1  dbl_ovrd=off
  Dual Port RAM : S-Function  AncestorBlock=xbsIndex_r3/Dual Port RAM  FunctionName=xldpram  Parameters=sfcn_mwsv__  mask(Xilinx Dual Port Random Access Memory){depth=2048, initVector=0, write_mode_A=Read After Write, write_mode_B=Read After Write, latency=4, mem_collision=off, init_zero=on, explicit_period=off, period=1, dbl_ovrd=off, rst_a=off, init_a=0, rst_b=off, init_b=0, show_param=off, distributed_mem=off, use_rpm=off, gen_core=off, xl_area=[0, 0, 0, 0, 0, 0, 0], xl_use_area=off}
      mask prompts: initVector "Initial Value Vector"; write_mode_A "Write Mode:  Port A"; write_mode_B "Write Mode:  Port B"; mem_collision "Provide Output Valid Port"; init_zero "Zero Initial Output  (otherwise NaN)"; explicit_period "Use Explicit Sample Period"; period "Sample Period  (use -1 to inherit first known input period)"; dbl_ovrd "Override with Doubles"; rst_a "Provide Reset Port for Port A Output Register"; init_a "Initial Value for Port A Output Register"; rst_b "Provide Reset Port for Port B Output Register"; init_b "Initial Value for Port B Output Register"; show_param "---------------------- Show Implementation Parameters -----------------------------------------------------------------------------------"; distributed_mem "Use Distributed Memory (instead of block RAM)"; use_rpm "Use Placement Information for Core"; gen_core "Generate Core"; xl_area "FPGA Area [Slices, FFs, BRAMs, LUTs, IOBs, Emb. Mults, TBUFs]"; xl_use_area "Use Area Above For Estimation"
      mask help: Dual port random access memory (RAM). Independent address, data and write enable ports allow shared access to a single memory space. Dual ports enable simultaneous access to the memory space at different sample rates using multiple data widths.
      mask init: same as poco_ref_al_r307/delay_wideband_prog0/delay_dp/Dual Port RAM
      mask Help: eval('xlWeb(xlhtmldoclink(''Dual Port RAM''))');
      mask StyleString: edit,edit,popup(Read After Write|Read Before Write|No Read On Write),popup(Read After Write|Read Before Write|No Read On Write),edit,checkbox,checkbox,checkbox,edit,checkbox,checkbox,edit,checkbox,edit,checkbox,checkbox,checkbox,checkbox,edit,checkbox
      mask CallbackString: |||||||xldpramCallback|||xldpramCallback||xldpramCallback||xldpramCallback|xldpramCallback||||
      mask Display:
      | patch([0 iWidth iWidth 0],[0 0 iHeight iHeight] ,bg);
      | patch([0 iWidth iWidth 0],[iCy-2 iCy-2 iCy+2 iCy+2] , .9* bg);
      | patch(logoX,logoY , fg);
      | port_label('input',1,'addr_A');
      | port_label('input',2,'data_A');
      | port_label('input',3,'we_A');
      | port_label('input',4,'addr_B');
      | port_label('input',dataBPNum,dataBStr);
      | port_label('input',weBPNum,weBStr);
      | port_label('input',rstAPNum,rstAStr);
      | port_label('input',rstBPNum,rstBStr);
      | port_label('output',1,'A');
      | port_label('output',doutBPNum,'B');
      | port_label('output',voutAPNum,voutAStr);
      | port_label('output',voutBPNum,voutBStr);
      | ;plot([0 0 iWidth iWidth 0], [0 iHeight iHeight 0 0]);
  wr_addr : xbsIndex_r3/Counter  cnt_type=Free Running  n_bits=11  bin_pt=0  arith_type=Unsigned  start_count=0  cnt_to=Inf  cnt_by_val=1  operation=Up  explicit_period=off  period=1  load_pin=off  rst=off  en=off  dbl_ovrd=off  show_param=off  use_rpm=on  gen_core=off
      settings: xl_area=[0, 0, 0, 0, 0, 0, 0]
  dout : Outport
  wires:
  Dual Port RAM/2 -> dout/1
  AddSub/1 -> Dual Port RAM/4
  delay/1 -> AddSub/2
  Constant4/1 -> Dual Port RAM/6
  din/1 -> Dual Port RAM/2, Dual Port RAM/5
  Constant2/1 -> Dual Port RAM/3
  wr_addr/1 -> Dual Port RAM/1, AddSub/1
